simulink model "vienna_car_part4"  (R2019b)
settings: Solver=ode23t  StartTime=0.0  StopTime=100  MaxStep=1e-4  RelTol=1e-4
values from neighbouring files (symbols this model uses):
  J = 0.01    [run.m]
  LM = 1.0122e-3    (= 0.0010122)    [run.m]    (also in run_to_complete.m)
  LMatrix = [LS 0 LM 0; 0 LS 0 LM; LM 0 LR 0; 0 LM 0 LR]    [run.m]    (also in run_to_complete.m)
  LR = lr + LM    (= 0.00107929)    [run.m]    (also in run_to_complete.m)
  pp = 2    [run.m]    (also in run_to_complete.m)
  RLInv = RMatrix/(LMatrix)    [run.m]    (also in run_to_complete.m)
  Rr = 2*5.10e-3    (= 0.0102)    [run.m]    (also in run_to_complete.m)
undefined symbols (not defined in the file or in its folder): air_density, drag_coefficient, equ_mass_of_rot_parts, gravity, mass, rolling_resistance_coefficient_0, rolling_resistance_coefficient_1, simulation_length_track, slope_of_track, surface_area, wheel_radius
libraries: simulink x3
settings Model: Creator=jamil  LastModifiedBy=jamil
settings SolverCC: ZeroCrossAlgorithm=Adaptive
settings DebuggingCC: IgnoredZcDiagnostic=none

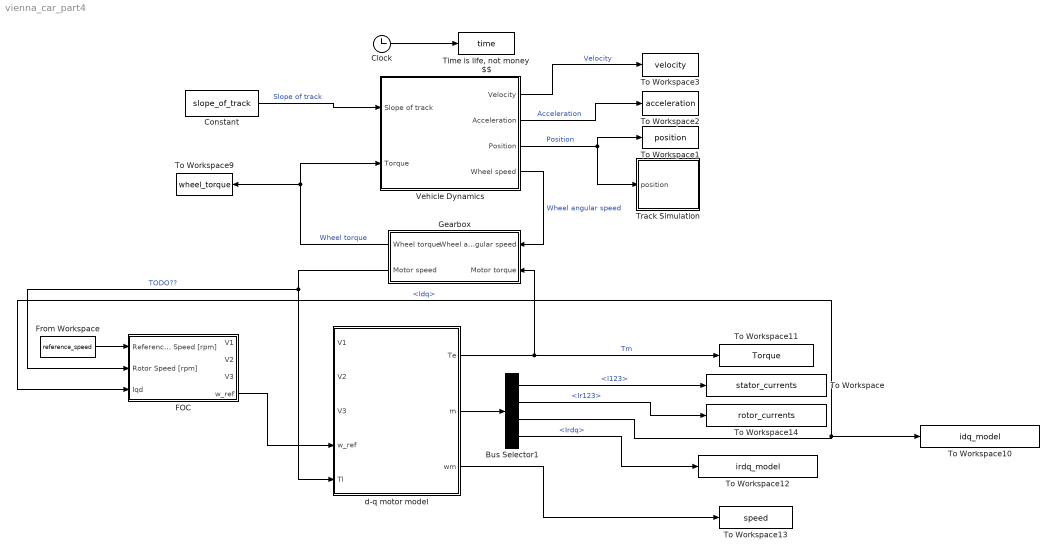
== system vienna_car_part4 ==
  Bus Selector1 : BusSelector  OutputSignals=I123,Ir123,Idq,Irdq
  Clock : Clock
  Constant : Constant  Value=slope_of_track
  FOC : Subsystem
  From Workspace : FromWorkspace  VariableName=reference_speed  SampleTime=0
  Gearbox : Subsystem
      mask Display: image('pics/gearbox_pic.jpg'); % Use "Edit Image" on toolstrip to change.
  "Time is life, not money $$" : ToWorkspace  VariableName=time  SampleTime=-1
  To Workspace : ToWorkspace  VariableName=stator_currents  SaveFormat=Timeseries  SampleTime=-1
  To Workspace1 : ToWorkspace  VariableName=position  SampleTime=-1
  To Workspace10 : ToWorkspace  VariableName=idq_model  SaveFormat=Timeseries  SampleTime=-1
  To Workspace11 : ToWorkspace  VariableName=Torque  SaveFormat=Timeseries  SampleTime=-1
  To Workspace12 : ToWorkspace  VariableName=irdq_model  SaveFormat=Timeseries  SampleTime=-1
  To Workspace13 : ToWorkspace  VariableName=speed  SaveFormat=Timeseries  SampleTime=-1
  To Workspace14 : ToWorkspace  VariableName=rotor_currents  SaveFormat=Timeseries  SampleTime=-1
  To Workspace2 : ToWorkspace  VariableName=acceleration  SampleTime=-1
  To Workspace3 : ToWorkspace  VariableName=velocity  SampleTime=-1
  To Workspace9 : ToWorkspace  VariableName=wheel_torque  SampleTime=-1
  Track Simulation : Subsystem
  Vehicle Dynamics : Subsystem
      mask Display: image('pics/car_dynamic_pic.jpg'); % Use "Edit Image" on toolstrip to change.
  d-q motor model : Subsystem
  wires:
  Vehicle Dynamics/2(Acceleration) -> To Workspace2/1  "Acceleration"
  Vehicle Dynamics/3(Position) -> Track Simulation/1(position), To Workspace1/1  "Position"
  Constant/1 -> Vehicle Dynamics/1("Slope of track ")  "Slope of track"
  Vehicle Dynamics/1(Velocity) -> To Workspace3/1  "Velocity"
  Clock/1 -> "Time is life, not money $$"/1
  Gearbox/2(Motor speed) -> d-q motor model/5(Tl), FOC/2(Rotor Speed [rpm])  "TODO??"
  From Workspace/1 -> FOC/1(Reference Speed [rpm])
  Vehicle Dynamics/4(Wheel speed) -> Gearbox/1(Wheel angular speed)  "Wheel angular speed"
  Gearbox/1("Wheel torque ") -> To Workspace9/1, Vehicle Dynamics/2(Torque)  "Wheel torque"
  d-q motor model/3(wm) -> To Workspace13/1
  Bus Selector1/3 -> FOC/3("Iqd "), To Workspace10/1  "<Idq>"
  d-q motor model/2(m) -> Bus Selector1/1
  Bus Selector1/2 -> To Workspace14/1  "<Ir123>"
  Bus Selector1/1 -> To Workspace/1  "<I123>"
  d-q motor model/1(Te) -> To Workspace11/1, Gearbox/2(Motor torque)  "Tm"
  Bus Selector1/4 -> To Workspace12/1  "<Irdq>"
  FOC/4(w_ref) -> d-q motor model/4(w_ref)

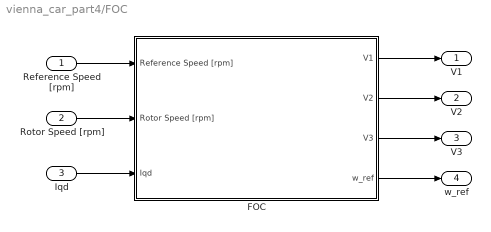
== system vienna_car_part4/FOC ==
  Reference Speed [rpm] : Inport
  Rotor Speed [rpm] : Inport  Port=2
  "Iqd " : Inport  Port=3
  "FOC " : Subsystem
  V1 : Outport
  V2 : Outport  Port=2
  V3 : Outport  Port=3
  w_ref : Outport  Port=4
  wires:
  Reference Speed [rpm]/1 -> "FOC "/1(Reference Speed [rpm])
  Rotor Speed [rpm]/1 -> "FOC "/2("Rotor Speed [rpm] ")
  "Iqd "/1 -> "FOC "/3("Iqd ")
  "FOC "/4(w_ref) -> w_ref/1
  "FOC "/1(V1) -> V1/1
  "FOC "/2(V2) -> V2/1
  "FOC "/3(V3) -> V3/1

== system vienna_car_part4/Gearbox ==
  Wheel angular speed : Inport
  Motor torque : Inport  Port=2
  Gain : Gain  Gain=8
  Gain1 : Gain  Gain=8
  "Wheel torque " : Outport
  Motor speed : Outport  Port=2
  wires:
  Gain/1 -> Motor speed/1
  Wheel angular speed/1 -> Gain/1
  Gain1/1 -> "Wheel torque "/1
  Motor torque/1 -> Gain1/1

== system vienna_car_part4/Track Simulation ==
  position : Inport
  Equal : RelationalOperator  OutDataTypeStr=boolean  RndMeth=Simplest
  Stop Simulation : Stop
  "Track " : Constant  Value=simulation_length_track
  wires:
  Equal/1 -> Stop Simulation/1
  position/1 -> Equal/1
  "Track "/1 -> Equal/2

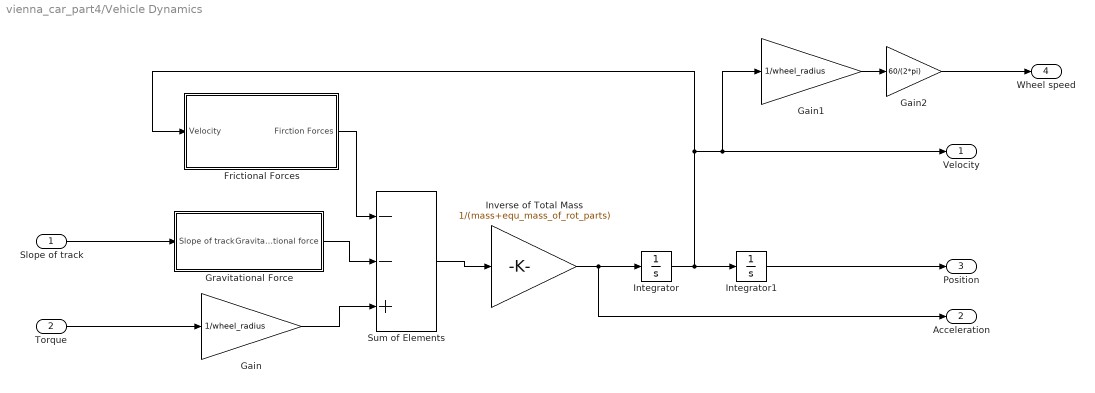
== system vienna_car_part4/Vehicle Dynamics ==
  "Slope of track " : Inport
  Torque : Inport  Port=2
  Frictional Forces : Subsystem
  Gain : Gain  Gain=1/wheel_radius
  Gain1 : Gain  Gain=1/wheel_radius
  Gain2 : Gain  Gain=60/(2*pi)
  Gravitational Force : Subsystem
  Integrator : Integrator
  Integrator1 : Integrator
  Inverse of Total Mass : Gain  Gain=1/(mass+equ_mass_of_rot_parts)
  Sum of Elements : Sum  Inputs=--+
  Velocity : Outport
  Acceleration : Outport  Port=2
  Position : Outport  Port=3
  Wheel speed : Outport  Port=4
  wires:
  Integrator1/1 -> Position/1
  Inverse of Total Mass/1 -> Integrator/1, Acceleration/1
  Sum of Elements/1 -> Inverse of Total Mass/1
  Frictional Forces/1(Firction Forces) -> Sum of Elements/1
  "Slope of track "/1 -> Gravitational Force/1(Slope of track)
  Gravitational Force/1(Gravitational force) -> Sum of Elements/2
  Torque/1 -> Gain/1
  Gain/1 -> Sum of Elements/3
  Gain2/1 -> Wheel speed/1
  Integrator/1 -> Frictional Forces/1(Velocity), Gain1/1, Velocity/1, Integrator1/1
  Gain1/1 -> Gain2/1

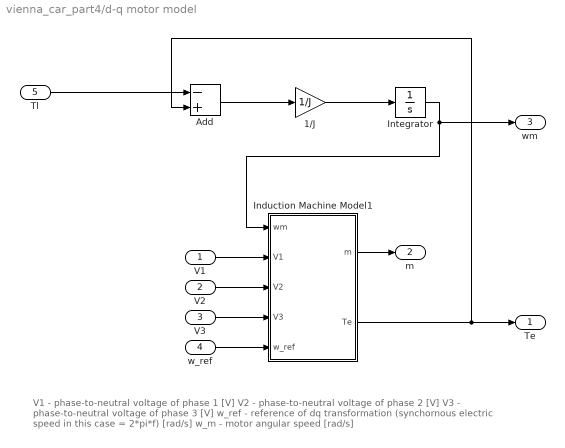
== system vienna_car_part4/d-q motor model ==
  note: V1 - phase-to-neutral voltage of phase 1 [V]
      | V2 - phase-to-neutral voltage of phase 2 [V]
      | V3 - phase-to-neutral voltage of phase 3 [V]
      | w_ref - reference of dq transformation (synchornous electric speed in this case = 2*pi*f) [rad/s]
      | w_m - motor angular speed [rad/s]
  V1 : Inport
  V2 : Inport  Port=2
  V3 : Inport  Port=3
  w_ref : Inport  Port=4
  Tl : Inport  Port=5
  1/J : Gain  Gain=1/J
  Add : Sum  Inputs=-+
  Induction Machine Model1 : Subsystem
  Integrator : Integrator
  Te : Outport  VectorParamsAs1DForOutWhenUnconnected=off
  m : Outport  Port=2  VectorParamsAs1DForOutWhenUnconnected=off
  wm : Outport  Port=3  VectorParamsAs1DForOutWhenUnconnected=off
  wires:
  Induction Machine Model1/1(m) -> m/1
  w_ref/1 -> Induction Machine Model1/5(w_ref)
  V1/1 -> Induction Machine Model1/2(V1)
  V2/1 -> Induction Machine Model1/3(V2)
  V3/1 -> Induction Machine Model1/4(V3)
  Integrator/1 -> Induction Machine Model1/1(wm), wm/1
  1/J/1 -> Integrator/1
  Add/1 -> 1/J/1
  Induction Machine Model1/2(Te) -> Add/2, Te/1
  Tl/1 -> Add/1

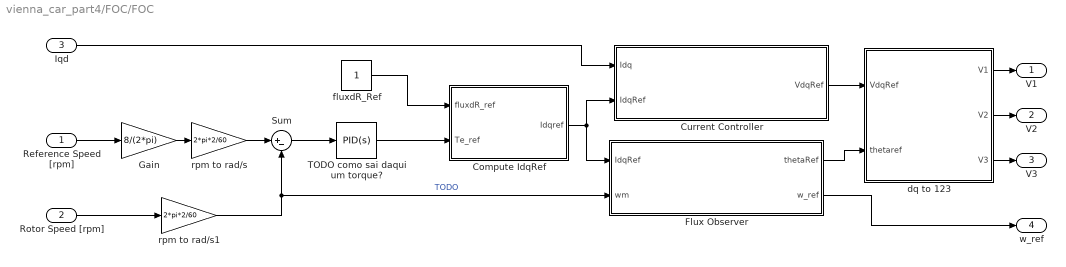
== system vienna_car_part4/FOC/FOC  ==
  Reference Speed [rpm] : Inport
  "Rotor Speed [rpm] " : Inport  Port=2
  "Iqd " : Inport  Port=3
  Compute IdqRef : Subsystem  TreatAsAtomicUnit=on
  "Current Controller " : Subsystem
  Flux Observer : Subsystem
  Gain : Gain  Gain=8/(2*pi)
  Sum : Sum  Inputs=|+-
  TODO como sai daqui um torque? : simulink/Continuous/PID Controller  Controller=PID  Form=Parallel  TimeDomain=Continuous-time  SampleTime=-1  IntegratorMethod=Forward Euler  FilterMethod=Forward Euler  ControllerParametersSource=internal  P=1  I=1  D=0  UseFilter=on  N=100  TunerSelectOption=Transfer Function Based (PID Tuner App)  InitialConditionSource=internal  InitialConditionForIntegrator=0  InitialConditionForFilter=0  DifferentiatorICPrevScaledInput=0  ExternalReset=none  TrackingMode=off  Kt=1  LimitOutput=off  UpperSaturationLimit=inf  LowerSaturationLimit=-inf  LinearizeAsGain=on  AntiWindupMode=none  Kb=1  POutMin=[]  POutMax=[]  IOutMin=[]  IOutMax=[]  DOutMin=[]  DOutMax=[]  NOutMin=[]  NOutMax=[]  SumOutMin=[]  SumOutMax=[]  SaturationOutMin=[]  SaturationOutMax=[]  PParamMin=[]  PParamMax=[]  IParamMin=[]  IParamMax=[]  DParamMin=[]  DParamMax=[]  NParamMin=[]  NParamMax=[]  KbParamMin=[]  KbParamMax=[]  KtParamMin=[]  KtParamMax=[]  KbOutMin=[]  KbOutMax=[]  KtOutMin=[]  KtOutMax=[]  IntegratorOutMin=[]  IntegratorOutMax=[]  FilterOutMin=[]  FilterOutMax=[]  SumI1OutMin=[]  SumI1OutMax=[]  SumI2OutMin=[]  SumI2OutMax=[]  SumI3OutMin=[]  SumI3OutMax=[]  SumI4OutMin=[]  SumI4OutMax=[]  SumDOutMin=[]  SumDOutMax=[]  DifferentiatorOutMin=[]  DifferentiatorOutMax=[]  FilterDiffOutCoefMin=[]  FilterDiffOutCoefMax=[]  ReciprocalOutMin=[]  ReciprocalOutMax=[]  SumDenOutMin=[]  SumDenOutMax=[]  SumNumOutMin=[]  SumNumOutMax=[]  DivideOutMin=[]  DivideOutMax=[]  IntegratorContinuousStateAttributes=''  IntegratorStateMustResolveToSignalObject=off  IntegratorRTWStateStorageClass=Auto  FilterContinuousStateAttributes=''  FilterStateMustResolveToSignalObject=off  FilterRTWStateStorageClass=Auto  ParallelPVariant=InternalParameters  IdealPVariant=Disabled  IVariant=InternalParameters  DVariant=InternalParameters  IntegratorVariant=Continuous  SatVariant=Disabled  AWVariant=Passthrough  PCopyVariant=Disabled  TRVariant=Disabled  FdbkBlocksVariant=Forward  IdealPFdbkVariant=Disabled  SatFdbkVariant=Disabled  DerivativeFilterVariant=ContFilter  NVariant=InternalParameters  NCopyVariant=Disabled  FilterICVariant=InternalICsFilter  IntegratorICVariant=InternalICs  ExternalResetVariant=Disabled  TRSumVariant=Passthrough  SumFdbkVariant=Disabled  SumVariant=Sum_PID
  dq to 123 : Subsystem
  "fluxdR_Ref " : Constant
  rpm to rad/s : Gain  Gain=2*pi*2/60
  rpm to rad/s1 : Gain  Gain=2*pi*2/60
  V1 : Outport
  V2 : Outport  Port=2
  V3 : Outport  Port=3
  w_ref : Outport  Port=4
  wires:
  "Rotor Speed [rpm] "/1 -> rpm to rad/s1/1
  Reference Speed [rpm]/1 -> Gain/1
  Gain/1 -> rpm to rad/s/1
  rpm to rad/s1/1 -> Flux Observer/2("wm "), Sum/2  "TODO"
  rpm to rad/s/1 -> Sum/1
  Sum/1 -> TODO como sai daqui um torque?/1
  "fluxdR_Ref "/1 -> Compute IdqRef/1(fluxdR_ref)
  TODO como sai daqui um torque?/1 -> Compute IdqRef/2(Te_ref)
  "Iqd "/1 -> "Current Controller "/1("Idq ")
  Compute IdqRef/1(Idqref) -> Flux Observer/1("IdqRef "), "Current Controller "/2("IdqRef ")
  Flux Observer/2(w_ref) -> w_ref/1
  dq to 123/1(V1) -> V1/1
  dq to 123/2(V2) -> V2/1
  dq to 123/3(V3) -> V3/1
  Flux Observer/1(thetaRef) -> dq to 123/2(thetaref)
  "Current Controller "/1("VdqRef ") -> dq to 123/1("VdqRef ")

== system vienna_car_part4/Vehicle Dynamics/Frictional Forces ==
  Velocity : Inport
  Constant : Constant  Value=mass*gravity
  Drag Coefficient Logic : Subsystem
  Drag Force : Constant  Value=0.5*air_density*surface_area*drag_coefficient
  If velocity negative invert signal : MATLAB Function  TreatAsAtomicUnit=on
  Product : Product  Inputs=3
  Sum of Friction Forces : Sum
  Firction Forces : Outport
  wires:
  Drag Force/1 -> Product/3
  Constant/1 -> Drag Coefficient Logic/1("Mass and Gravity ")
  Drag Coefficient Logic/1(Friction Force) -> Sum of Friction Forces/1
  Velocity/1 -> Product/1, Product/2, If velocity negative invert signal/2(velocity), Drag Coefficient Logic/2(Velocity)
  Product/1 -> Sum of Friction Forces/2
  Sum of Friction Forces/1 -> If velocity negative invert signal/1(u)
  If velocity negative invert signal/1(y) -> Firction Forces/1

== system vienna_car_part4/Vehicle Dynamics/Gravitational Force ==
  Slope of track : Inport
  Constant : Constant  Value=mass*gravity
  Degree to Radians : Gain  Gain=2*pi/360
  Product1 : Product
  Trigonometric Function : Trigonometry
  Gravitational force : Outport
  wires:
  Product1/1 -> Gravitational force/1
  Constant/1 -> Product1/1
  Trigonometric Function/1 -> Product1/2
  Slope of track/1 -> Degree to Radians/1
  Degree to Radians/1 -> Trigonometric Function/1

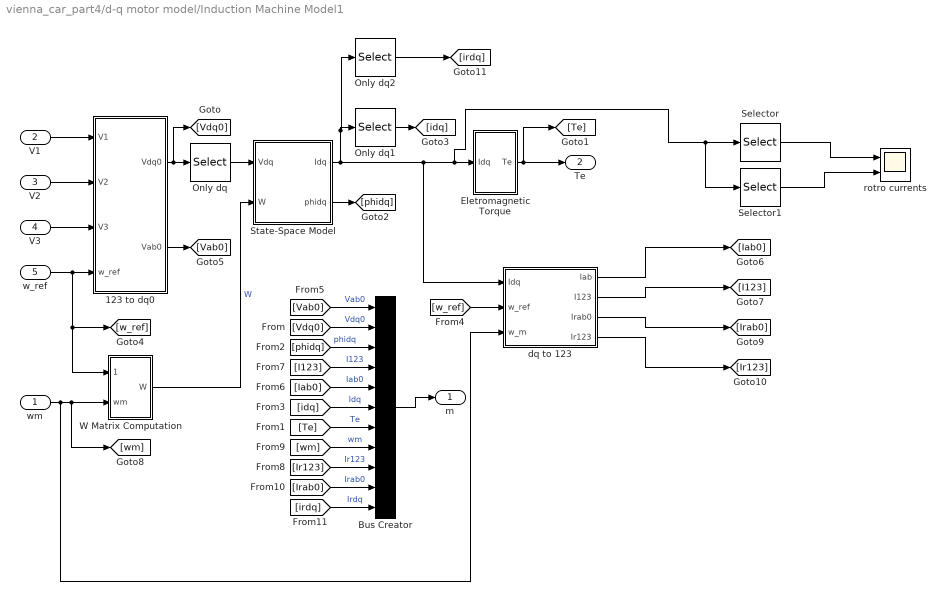
== system vienna_car_part4/d-q motor model/Induction Machine Model1 ==
  wm : Inport
  V1 : Inport  Port=2
  V2 : Inport  Port=3
  V3 : Inport  Port=4
  w_ref : Inport  Port=5
  123 to dq0 : Subsystem
  Bus Creator : BusCreator  Inputs=11
  Eletromagnetic Torque : Subsystem
  Only dq : Selector  InputPortWidth=3  IndexOptions=Index vector (dialog)  Indices=[1 2]  OutputSizes=1
  Only dq1 : Selector  InputPortWidth=4  IndexOptions=Index vector (dialog)  Indices=[1 2]  OutputSizes=1
  Only dq2 : Selector  InputPortWidth=4  IndexOptions=Index vector (dialog)  Indices=[3 4]  OutputSizes=1
  Selector : Selector  InputPortWidth=4  IndexOptions=Index vector (dialog)  Indices=[1 2]  OutputSizes=1
  Selector1 : Selector  InputPortWidth=4  IndexOptions=Index vector (dialog)  Indices=[3 4]  OutputSizes=1
  State-Space Model : Subsystem
  W Matrix Computation : Subsystem
  dq to 123 : Subsystem
  rotro currents : Scope  NumInputPorts=2
  m : Outport  VectorParamsAs1DForOutWhenUnconnected=off
  Te : Outport  Port=2  VectorParamsAs1DForOutWhenUnconnected=off
  wires:
  123 to dq0/1(Vdq0) -> Only dq/1, [Vdq0]
  V3/1 -> 123 to dq0/3(V3)
  V2/1 -> 123 to dq0/2(V2)
  wm/1 -> dq to 123/3(w_m), [wm], W Matrix Computation/2(wm)
  123 to dq0/2(Vab0) -> [Vab0]
  W Matrix Computation/1(W) -> State-Space Model/2(W)  "W"
  Only dq/1 -> State-Space Model/1(Vdq)
  Eletromagnetic Torque/1(Te) -> Te/1, [Te]
  V1/1 -> 123 to dq0/1(V1)
  [w_ref] -> dq to 123/2(w_ref)
  State-Space Model/2(phidq) -> [phidq]
  dq to 123/1(Iab) -> [Iab0]
  dq to 123/2(I123) -> [I123]
  [Vab0] -> Bus Creator/1  "Vab0"
  [Vdq0] -> Bus Creator/2  "Vdq0"
  [phidq] -> Bus Creator/3  "phidq"
  [I123] -> Bus Creator/4  "I123"
  [Iab0] -> Bus Creator/5  "Iab0"
  [idq] -> Bus Creator/6  "Idq"
  [Te] -> Bus Creator/7  "Te"
  Bus Creator/1 -> m/1
  Only dq1/1 -> [idq]
  w_ref/1 -> 123 to dq0/4(w_ref), W Matrix Computation/1(w_ref), [w_ref]
  [wm] -> Bus Creator/8  "wm"
  dq to 123/4(Ir123) -> [Ir123]
  dq to 123/3(Irab0) -> [Irab0]
  [Ir123] -> Bus Creator/9  "Ir123"
  [Irab0] -> Bus Creator/10  "Irab0"
  Selector/1 -> rotro currents/1
  Selector1/1 -> rotro currents/2
  State-Space Model/1(Idq) -> dq to 123/1(Idq), Selector1/1, Selector/1, Eletromagnetic Torque/1(Idq), Only dq2/1, Only dq1/1
  Only dq2/1 -> [irdq]
  [irdq] -> Bus Creator/11  "Irdq"

== system vienna_car_part4/FOC/FOC /Compute IdqRef ==
  fluxdR_ref : Inport
  Te_ref : Inport  Port=2
  Bus Creator : BusCreator  Inputs=2
  Divide : Product  Inputs=*/
  Gain : Gain  Gain=(2/3)*(1/pp)*(LR/LM)
  Gain1 : Gain  Gain=1/LM
  Idqref : Outport
  wires:
  Te_ref/1 -> Divide/1
  fluxdR_ref/1 -> Divide/2, Gain1/1
  Divide/1 -> Gain/1
  Gain1/1 -> Bus Creator/1  "id"
  Gain/1 -> Bus Creator/2  "iq"
  Bus Creator/1 -> Idqref/1

== system vienna_car_part4/FOC/FOC /Current Controller  ==
  "Idq " : Inport
  "IdqRef " : Inport  Port=2
  Bus Creator : BusCreator  Inputs=2
  Bus Selector : BusSelector  OutputSignals=signal1,signal2
  Sum : Sum  Inputs=|+-
  TODO : simulink/Continuous/PID Controller  Controller=PID  Form=Parallel  TimeDomain=Continuous-time  SampleTime=-1  IntegratorMethod=Forward Euler  FilterMethod=Forward Euler  ControllerParametersSource=internal  P=1  I=1  D=0  UseFilter=on  N=100  TunerSelectOption=Transfer Function Based (PID Tuner App)  InitialConditionSource=internal  InitialConditionForIntegrator=0  InitialConditionForFilter=0  DifferentiatorICPrevScaledInput=0  ExternalReset=none  TrackingMode=off  Kt=1  LimitOutput=off  UpperSaturationLimit=inf  LowerSaturationLimit=-inf  LinearizeAsGain=on  AntiWindupMode=none  Kb=1  POutMin=[]  POutMax=[]  IOutMin=[]  IOutMax=[]  DOutMin=[]  DOutMax=[]  NOutMin=[]  NOutMax=[]  SumOutMin=[]  SumOutMax=[]  SaturationOutMin=[]  SaturationOutMax=[]  PParamMin=[]  PParamMax=[]  IParamMin=[]  IParamMax=[]  DParamMin=[]  DParamMax=[]  NParamMin=[]  NParamMax=[]  KbParamMin=[]  KbParamMax=[]  KtParamMin=[]  KtParamMax=[]  KbOutMin=[]  KbOutMax=[]  KtOutMin=[]  KtOutMax=[]  IntegratorOutMin=[]  IntegratorOutMax=[]  FilterOutMin=[]  FilterOutMax=[]  SumI1OutMin=[]  SumI1OutMax=[]  SumI2OutMin=[]  SumI2OutMax=[]  SumI3OutMin=[]  SumI3OutMax=[]  SumI4OutMin=[]  SumI4OutMax=[]  SumDOutMin=[]  SumDOutMax=[]  DifferentiatorOutMin=[]  DifferentiatorOutMax=[]  FilterDiffOutCoefMin=[]  FilterDiffOutCoefMax=[]  ReciprocalOutMin=[]  ReciprocalOutMax=[]  SumDenOutMin=[]  SumDenOutMax=[]  SumNumOutMin=[]  SumNumOutMax=[]  DivideOutMin=[]  DivideOutMax=[]  IntegratorContinuousStateAttributes=''  IntegratorStateMustResolveToSignalObject=off  IntegratorRTWStateStorageClass=Auto  FilterContinuousStateAttributes=''  FilterStateMustResolveToSignalObject=off  FilterRTWStateStorageClass=Auto  ParallelPVariant=InternalParameters  IdealPVariant=Disabled  IVariant=InternalParameters  DVariant=InternalParameters  IntegratorVariant=Continuous  SatVariant=Disabled  AWVariant=Passthrough  PCopyVariant=Disabled  TRVariant=Disabled  FdbkBlocksVariant=Forward  IdealPFdbkVariant=Disabled  SatFdbkVariant=Disabled  DerivativeFilterVariant=ContFilter  NVariant=InternalParameters  NCopyVariant=Disabled  FilterICVariant=InternalICsFilter  IntegratorICVariant=InternalICs  ExternalResetVariant=Disabled  TRSumVariant=Passthrough  SumFdbkVariant=Disabled  SumVariant=Sum_PID
  "TODO1 " : simulink/Continuous/PID Controller  Controller=PID  Form=Parallel  TimeDomain=Continuous-time  SampleTime=-1  IntegratorMethod=Forward Euler  FilterMethod=Forward Euler  ControllerParametersSource=internal  P=1  I=1  D=0  UseFilter=on  N=100  TunerSelectOption=Transfer Function Based (PID Tuner App)  InitialConditionSource=internal  InitialConditionForIntegrator=0  InitialConditionForFilter=0  DifferentiatorICPrevScaledInput=0  ExternalReset=none  TrackingMode=off  Kt=1  LimitOutput=off  UpperSaturationLimit=inf  LowerSaturationLimit=-inf  LinearizeAsGain=on  AntiWindupMode=none  Kb=1  POutMin=[]  POutMax=[]  IOutMin=[]  IOutMax=[]  DOutMin=[]  DOutMax=[]  NOutMin=[]  NOutMax=[]  SumOutMin=[]  SumOutMax=[]  SaturationOutMin=[]  SaturationOutMax=[]  PParamMin=[]  PParamMax=[]  IParamMin=[]  IParamMax=[]  DParamMin=[]  DParamMax=[]  NParamMin=[]  NParamMax=[]  KbParamMin=[]  KbParamMax=[]  KtParamMin=[]  KtParamMax=[]  KbOutMin=[]  KbOutMax=[]  KtOutMin=[]  KtOutMax=[]  IntegratorOutMin=[]  IntegratorOutMax=[]  FilterOutMin=[]  FilterOutMax=[]  SumI1OutMin=[]  SumI1OutMax=[]  SumI2OutMin=[]  SumI2OutMax=[]  SumI3OutMin=[]  SumI3OutMax=[]  SumI4OutMin=[]  SumI4OutMax=[]  SumDOutMin=[]  SumDOutMax=[]  DifferentiatorOutMin=[]  DifferentiatorOutMax=[]  FilterDiffOutCoefMin=[]  FilterDiffOutCoefMax=[]  ReciprocalOutMin=[]  ReciprocalOutMax=[]  SumDenOutMin=[]  SumDenOutMax=[]  SumNumOutMin=[]  SumNumOutMax=[]  DivideOutMin=[]  DivideOutMax=[]  IntegratorContinuousStateAttributes=''  IntegratorStateMustResolveToSignalObject=off  IntegratorRTWStateStorageClass=Auto  FilterContinuousStateAttributes=''  FilterStateMustResolveToSignalObject=off  FilterRTWStateStorageClass=Auto  ParallelPVariant=InternalParameters  IdealPVariant=Disabled  IVariant=InternalParameters  DVariant=InternalParameters  IntegratorVariant=Continuous  SatVariant=Disabled  AWVariant=Passthrough  PCopyVariant=Disabled  TRVariant=Disabled  FdbkBlocksVariant=Forward  IdealPFdbkVariant=Disabled  SatFdbkVariant=Disabled  DerivativeFilterVariant=ContFilter  NVariant=InternalParameters  NCopyVariant=Disabled  FilterICVariant=InternalICsFilter  IntegratorICVariant=InternalICs  ExternalResetVariant=Disabled  TRSumVariant=Passthrough  SumFdbkVariant=Disabled  SumVariant=Sum_PID
  "VdqRef " : Outport
  wires:
  "IdqRef "/1 -> Sum/1
  "Idq "/1 -> Sum/2
  Sum/1 -> Bus Selector/1
  Bus Selector/2 -> TODO/1  "<signal2>"
  Bus Selector/1 -> "TODO1 "/1  "<signal1>"
  Bus Creator/1 -> "VdqRef "/1
  "TODO1 "/1 -> Bus Creator/1
  TODO/1 -> Bus Creator/2

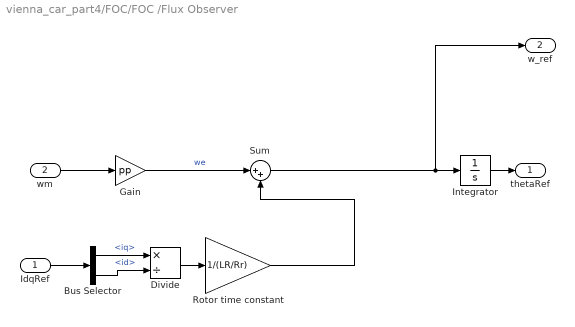
== system vienna_car_part4/FOC/FOC /Flux Observer ==
  "IdqRef " : Inport
  "wm " : Inport  Port=2
  Bus Selector : BusSelector  OutputSignals=iq,id
  Divide : Product  Inputs=*/
  Gain : Gain  Gain=pp
  Integrator : Integrator
  Rotor time constant : Gain  Gain=1/(LR/Rr)
  Sum : Sum  Inputs=|++
  thetaRef : Outport
  w_ref : Outport  Port=2
  wires:
  "wm "/1 -> Gain/1
  Gain/1 -> Sum/1  "we"
  "IdqRef "/1 -> Bus Selector/1
  Sum/1 -> w_ref/1, Integrator/1
  Integrator/1 -> thetaRef/1
  Bus Selector/1 -> Divide/1  "<iq>"
  Bus Selector/2 -> Divide/2  "<id>"
  Divide/1 -> Rotor time constant/1
  Rotor time constant/1 -> Sum/2

== system vienna_car_part4/FOC/FOC /dq to 123 ==
  "VdqRef " : Inport
  thetaref : Inport  Port=2
  V1 : Outport
  V2 : Outport  Port=2
  V3 : Outport  Port=3

== system vienna_car_part4/Vehicle Dynamics/Frictional Forces/Drag Coefficient Logic ==
  "Mass and Gravity " : Inport
  Velocity : Inport  Port=2
  If : If  IfExpression=u1 > 0.01
  If Action Subsystem : Subsystem  TreatAsAtomicUnit=on
  If Action Subsystem1 : Subsystem  TreatAsAtomicUnit=on
  Merge : Merge
  Friction Force : Outport
  wires:
  If Action Subsystem/1(Out1) -> Merge/2
  If Action Subsystem1/1(Out1) -> Merge/1
  If/2 -> If Action Subsystem1/Action
  "Mass and Gravity "/1 -> If Action Subsystem/1(In1), If Action Subsystem1/1(In1)
  Merge/1 -> Friction Force/1
  If/1 -> If Action Subsystem/Action
  Velocity/1 -> If/1

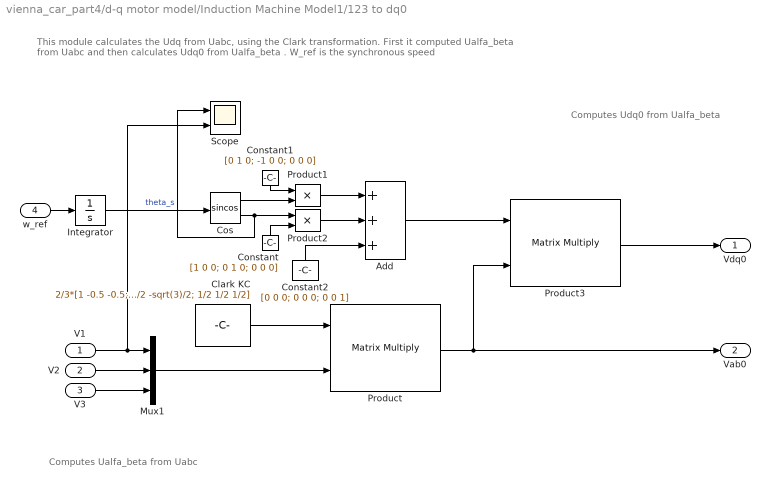
== system vienna_car_part4/d-q motor model/Induction Machine Model1/123 to dq0 ==
  note: Computes Ualfa_beta from Uabc
  note: This module calculates the Udq from Uabc, using the Clark transformation.
      | First it computed Ualfa_beta from Uabc and then calculates Udq0 from Ualfa_beta .
      | W_ref is the synchronous speed
  note: Computes Udq0 from Ualfa_beta
  V1 : Inport
  V2 : Inport  Port=2
  V3 : Inport  Port=3
  w_ref : Inport  Port=4
  Add : Sum  Inputs=+++
  Clark KC : Constant  Value=2/3*[1 -0.5 -0.5; 0 sqrt(3)/2 -sqrt(3)/2; 1/2 1/2 1/2]
  Constant : Constant  Value=[1 0 0; 0 1 0; 0 0 0]
  Constant1 : Constant  Value=[0 1 0; -1 0 0; 0 0 0]
  Constant2 : Constant  Value=[0 0 0; 0 0 0; 0 0 1]
  Cos : Trigonometry  Operator=sincos
  Integrator : Integrator
  Mux1 : Mux  Inputs=3
  Product : Product  Multiplication=Matrix(*)
  Product1 : Product
  Product2 : Product
  Product3 : Product  Multiplication=Matrix(*)
  Scope : Scope  NumInputPorts=2
  Vdq0 : Outport  VectorParamsAs1DForOutWhenUnconnected=off
  Vab0 : Outport  Port=2  VectorParamsAs1DForOutWhenUnconnected=off
  wires:
  Clark KC/1 -> Product/1
  Mux1/1 -> Product/2
  Product/1 -> Product3/2, Vab0/1
  Integrator/1 -> Cos/1  "theta_s"
  Cos/1 -> Product1/2
  Constant1/1 -> Product1/1
  Cos/2 -> Scope/1, Product2/1
  Constant/1 -> Product2/2
  Product1/1 -> Add/1
  Product2/1 -> Add/2
  Add/1 -> Product3/1
  Product3/1 -> Vdq0/1
  w_ref/1 -> Integrator/1
  Constant2/1 -> Add/3
  V2/1 -> Mux1/2
  V3/1 -> Mux1/3
  V1/1 -> Mux1/1, Scope/2

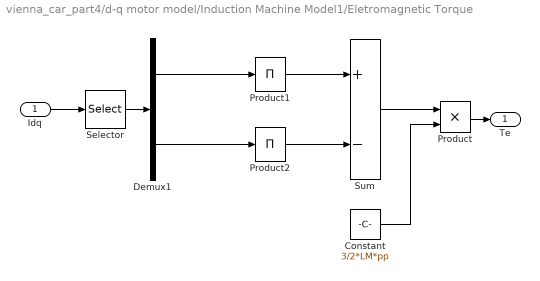
== system vienna_car_part4/d-q motor model/Induction Machine Model1/Eletromagnetic Torque ==
  Idq : Inport
  Constant : Constant  Value=3/2*LM*pp
  Demux1 : Demux  Outputs=2
  Product : Product
  Product1 : Product  Inputs=1
  Product2 : Product  Inputs=1
  Selector : Selector  InputPortWidth=4  IndexOptions=Index vector (dialog)  Indices=[2 3 1 4]  OutputSizes=1
  Sum : Sum  Inputs=+-
  Te : Outport  VectorParamsAs1DForOutWhenUnconnected=off
  wires:
  Sum/1 -> Product/1
  Product1/1 -> Sum/1
  Demux1/1 -> Product1/1
  Product2/1 -> Sum/2
  Constant/1 -> Product/2
  Demux1/2 -> Product2/1
  Product/1 -> Te/1
  Idq/1 -> Selector/1
  Selector/1 -> Demux1/1

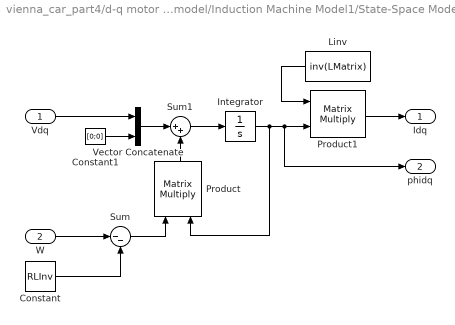
== system vienna_car_part4/d-q motor model/Induction Machine Model1/State-Space Model ==
  Vdq : Inport
  W : Inport  Port=2
  Constant : Constant  Value=RLInv  VectorParams1D=off
  Constant1 : Constant  Value=[0;0]
  Integrator : Integrator
  Linv : Constant  Value=inv(LMatrix)  VectorParams1D=off
  Product : Product  Multiplication=Matrix(*)
  Product1 : Product  Multiplication=Matrix(*)
  Sum : Sum  Inputs=|--
  Sum1 : Sum  Inputs=|++
  Vector Concatenate : Concatenate
  Idq : Outport  VectorParamsAs1DForOutWhenUnconnected=off
  phidq : Outport  Port=2  VectorParamsAs1DForOutWhenUnconnected=off
  wires:
  W/1 -> Sum/1
  Product/1 -> Sum1/2
  Constant/1 -> Sum/2
  Integrator/1 -> phidq/1, Product1/2, Product/2
  Product1/1 -> Idq/1
  Sum1/1 -> Integrator/1
  Sum/1 -> Product/1
  Linv/1 -> Product1/1
  Vdq/1 -> Vector Concatenate/1
  Constant1/1 -> Vector Concatenate/2
  Vector Concatenate/1 -> Sum1/1

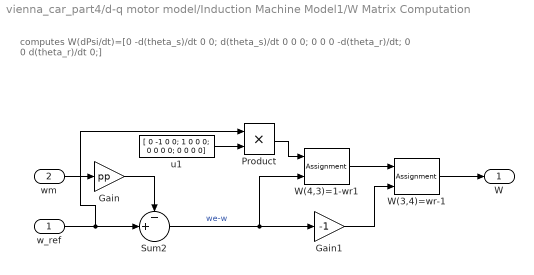
== system vienna_car_part4/d-q motor model/Induction Machine Model1/W Matrix Computation ==
  note: computes W(dPsi/dt)=[0                     -d(theta_s)/dt          0                       0;
      |                                     d(theta_s)/dt           0                      0                      0;
      |                                    0                              0                      0             -d(theta_r)/dt;
      |                                    0                              0             d(theta_r)/dt              0;]
  w_ref : Inport
  wm : Inport  Port=2
  Gain : Gain  Gain=pp
  Gain1 : Gain  Gain=-1  SaturateOnIntegerOverflow=on  OutDataTypeStr=Inherit: Same as input  ParamDataTypeStr=Inherit: Same as input
  Product : Product
  Sum2 : Sum  Inputs=-+|  SaturateOnIntegerOverflow=on  InputSameDT=on  OutDataTypeStr=Inherit: Same as first input
  W(3,4)=wr-1 : Assignment  NumberOfDimensions=2  IndexOptions=Index vector (dialog),Index vector (dialog)  Indices=3,4  OutputSizes=1,1
  W(4,3)=1-wr1 : Assignment  NumberOfDimensions=2  IndexOptions=Index vector (dialog),Index vector (dialog)  Indices=4,3  OutputSizes=1,1
  u1 : Constant  Value="[ 0 -1  0  0; 1  0  0  0;  0  0  0  0;  0  0  0  0]"
  W : Outport  InitialOutput=0  VectorParamsAs1DForOutWhenUnconnected=off
  wires:
  Gain1/1 -> W(3,4)=wr-1/2
  W(3,4)=wr-1/1 -> W/1
  Sum2/1 -> W(4,3)=1-wr1/2, Gain1/1  "we-w"
  wm/1 -> Gain/1
  W(4,3)=1-wr1/1 -> W(3,4)=wr-1/1
  Gain/1 -> Sum2/1
  w_ref/1 -> Product/1, Sum2/2
  u1/1 -> Product/2
  Product/1 -> W(4,3)=1-wr1/1

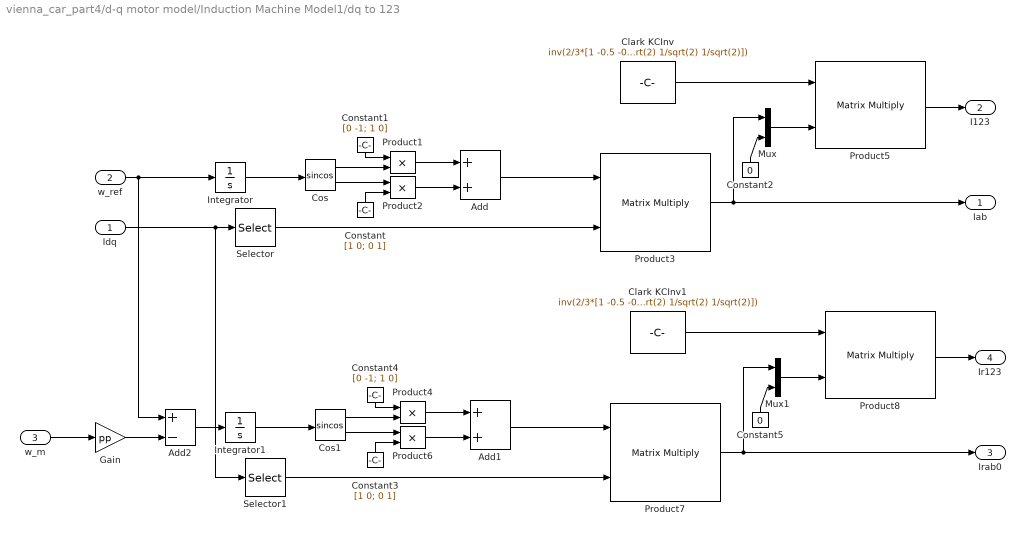
== system vienna_car_part4/d-q motor model/Induction Machine Model1/dq to 123 ==
  Idq : Inport
  w_ref : Inport  Port=2
  w_m : Inport  Port=3
  Add : Sum
  Add1 : Sum
  Add2 : Sum  Inputs=+-
  Clark KCInv : Constant  Value=inv(2/3*[1 -0.5 -0.5; 0 sqrt(3)/2 -sqrt(3)/2; 1/sqrt(2) 1/sqrt(2) 1/sqrt(2)])
  Clark KCInv1 : Constant  Value=inv(2/3*[1 -0.5 -0.5; 0 sqrt(3)/2 -sqrt(3)/2; 1/sqrt(2) 1/sqrt(2) 1/sqrt(2)])
  Constant : Constant  Value=[1 0; 0 1]
  Constant1 : Constant  Value=[0 -1; 1 0]
  Constant2 : Constant  Value=0
  Constant3 : Constant  Value=[1 0; 0 1]
  Constant4 : Constant  Value=[0 -1; 1 0]
  Constant5 : Constant  Value=0
  Cos : Trigonometry  Operator=sincos
  Cos1 : Trigonometry  Operator=sincos
  Gain : Gain  Gain=pp
  Integrator : Integrator
  Integrator1 : Integrator
  Mux : Mux  Inputs=2
  Mux1 : Mux  Inputs=2
  Product{1..2,4,6} (4 alike) : Product
  Product{3,5,7..8} (4 alike) : Product  Multiplication=Matrix(*)
  Selector : Selector  InputPortWidth=4  IndexOptions=Index vector (dialog)  Indices=[1 2]  OutputSizes=1
  Selector1 : Selector  InputPortWidth=4  IndexOptions=Index vector (dialog)  Indices=[3 4]  OutputSizes=1
  Iab : Outport  VectorParamsAs1DForOutWhenUnconnected=off
  I123 : Outport  Port=2  VectorParamsAs1DForOutWhenUnconnected=off
  Irab0 : Outport  Port=3  VectorParamsAs1DForOutWhenUnconnected=off
  Ir123 : Outport  Port=4  VectorParamsAs1DForOutWhenUnconnected=off
  wires:
  Cos/1 -> Product1/2
  Constant1/1 -> Product1/1
  Product2/1 -> Add/2
  Cos/2 -> Product2/1
  Product1/1 -> Add/1
  Constant/1 -> Product2/2
  Add/1 -> Product3/1
  Product3/1 -> Mux/1, Iab/1
  Clark KCInv/1 -> Product5/1
  Product5/1 -> I123/1
  Mux/1 -> Product5/2
  Constant2/1 -> Mux/2
  Selector/1 -> Product3/2
  Integrator/1 -> Cos/1
  w_ref/1 -> Integrator/1, Add2/1
  Cos1/1 -> Product4/2
  Selector1/1 -> Product7/2
  Integrator1/1 -> Cos1/1
  Clark KCInv1/1 -> Product8/1
  Constant3/1 -> Product6/2
  Product8/1 -> Ir123/1
  Idq/1 -> Selector1/1, Selector/1
  Cos1/2 -> Product6/1
  Constant4/1 -> Product4/1
  Constant5/1 -> Mux1/2
  Product4/1 -> Add1/1
  Add1/1 -> Product7/1
  Mux1/1 -> Product8/2
  Product6/1 -> Add1/2
  Product7/1 -> Mux1/1, Irab0/1
  w_m/1 -> Gain/1
  Add2/1 -> Integrator1/1
  Gain/1 -> Add2/2

== system vienna_car_part4/Vehicle Dynamics/Frictional Forces/Drag Coefficient Logic/If Action Subsystem ==
  In1 : Inport
  Action Port : ActionPort  ActionPortLabel=if(u1 > 0.01)
  Gain : Gain  Gain=rolling_resistance_coefficient_1
  Out1 : Outport
  wires:
  In1/1 -> Gain/1
  Gain/1 -> Out1/1

== system vienna_car_part4/Vehicle Dynamics/Frictional Forces/Drag Coefficient Logic/If Action Subsystem1 ==
  In1 : Inport
  Action Port : ActionPort  ActionPortLabel=else
  Gain : Gain  Gain=rolling_resistance_coefficient_0
  Out1 : Outport
  wires:
  In1/1 -> Gain/1
  Gain/1 -> Out1/1

== matlab function vienna_car_part4/Vehicle Dynamics/Frictional Forces/If velocity negative invert signal ==
  data: u input; y output; velocity input
function y = fcn(u, velocity)
if (velocity < 0 )
    y = - u;
else
    y = u;
end
end
